simulink model "B4CostaTest"  (R2022a)
settings: Solver=VariableStepAuto  StartTime=0.0  StopTime=40  RelTol=1e-4  AbsTol=1e-4
values from neighbouring files (symbols this model uses):
  AinfK_h_B4 = -23    [B4.m]
  AinfK_p_B4 = 1.0    (= 1)    [B4.m]
  AinfK_s_B4 = 9.0    (= 9)    [B4.m]
  AinfNa_h_B4 = -37    [B4.m]
  AinfNa_p_B4 = 1.0    (= 1)    [B4.m]
  AinfNa_s_B4 = 5.0    (= 5)    [B4.m]
  AK_B4_0 = 0.4    [B4.m]
  ANa_B4_0 = 0.4    [B4.m]
  BinfNa_h_B4 = -43.0    (= -43)    [B4.m]
  BinfNa_p_B4 = 1.0    (= 1)    [B4.m]
  BinfNa_s_B4 = 5.0    (= 5)    [B4.m]
  BNa_B4_0 = 0.4    [B4.m]
  Cm_B4 = 0.01    [B4.m]    (also in CtrlParaSNSTuning.m)
  EK_B4 = -70    [B4.m]
  EL_B4 = -60    [B4.m]    (also in CtrlParaSNSTuning.m)
  ENa_B4 = 30    [B4.m]
  gK_B4 = 12    [B4.m]
  gL_B4 = 0.1    [B4.m]    (also in CtrlParaSNSTuning.m = 0.2008)
  gNa_B4 = 25    [B4.m]
  pK_B4 = 4    [B4.m]
  pNa_B4 = 3    [B4.m]
  RK_B4 = 0    [B4.m]
  RL_B4 = 0    [B4.m]    (also in CtrlParaSNSTuning.m)
  RNa_B4 = 0    [B4.m]
  spikedur_B4 = 0.003    [B4.m]
  tAK_h_B4 = -8.0    (= -8)    [B4.m]
  tAK_p_B4 = 1.0    (= 1)    [B4.m]
  tAK_s_B4 = 10.0    (= 10)    [B4.m]
  tAK_tmax_B4 = 0.04    [B4.m]
  tAK_tmin_B4 = 0.004    [B4.m]
  tANa_h_B4 = -43    [B4.m]
  tANa_p_B4 = 1.0    (= 1)    [B4.m]
  tANa_s_B4 = 4.0    (= 4)    [B4.m]
  tANa_tmax_B4 = 0.006    [B4.m]
  tANa_tmin_B4 = 0.001    [B4.m]
  tBNa_h_B4 = -38    [B4.m]
  tBNa_p_B4 = 1.0    (= 1)    [B4.m]
  tBNa_s_B4 = 10.0    (= 10)    [B4.m]
  tBNa_tmax_B4 = 0.02    [B4.m]
  tBNa_tmin_B4 = 0.005    [B4.m]
  V_B4_0 = -60    [B4.m]    (also in CtrlParaSNSTuning.m; InitPara.m)
undefined symbols (not defined in the file or in its folder): Iapp
libraries: simulink x1
settings Model: Creator=liyan  LastModifiedBy=liyan

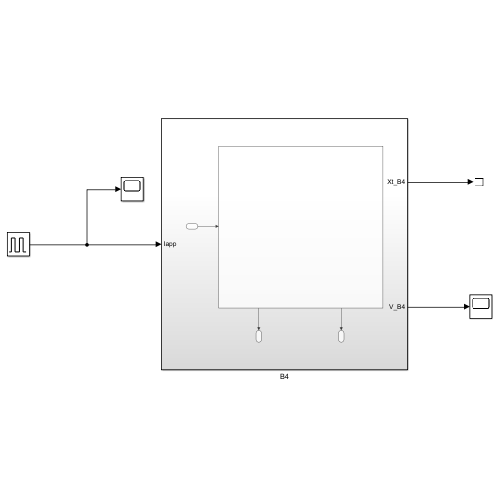
[thumbnail: Simulink's stored preview of the top-level diagram]
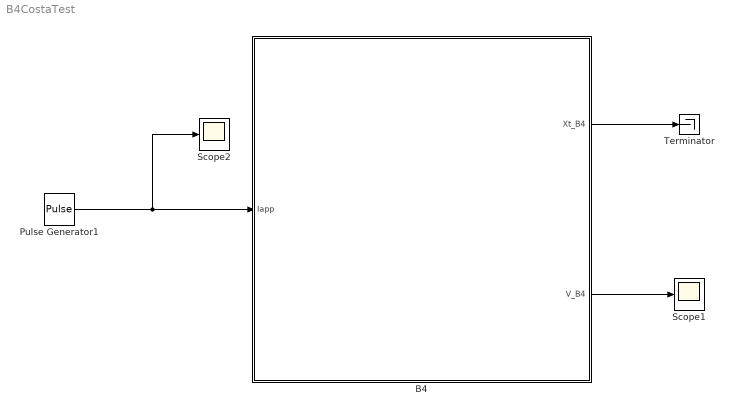
== system B4CostaTest ==
  B4 : Subsystem
  Pulse Generator1 : DiscretePulseGenerator  PulseType=Time based  Amplitude=Iapp  Period=40  PulseWidth=0.3/40*100  PhaseDelay=30
  Scope1 : Scope
  Scope2 : Scope
  Terminator : Terminator
  wires:
  Pulse Generator1/1 -> B4/1(Iapp), Scope2/1
  B4/2(V_B4) -> Scope1/1
  B4/1(Xt_B4) -> Terminator/1

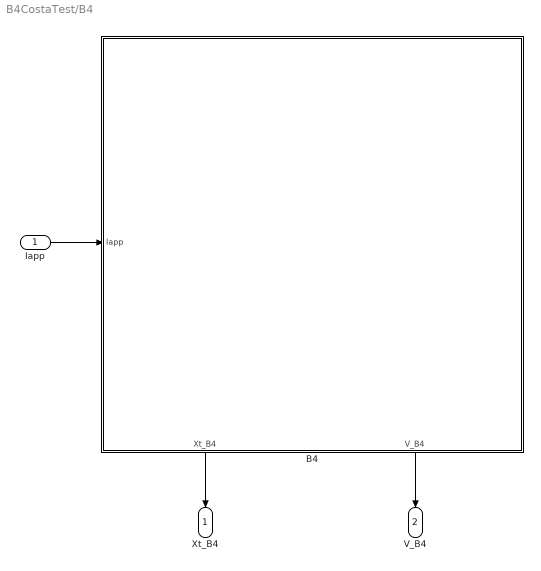
== system B4CostaTest/B4 ==
  Iapp : Inport
  B4 : Subsystem
      settings: PortSchema="{\"entries\":[{\"content\":{\"sides\":[{\"content\":{\"connectorIds\":[\"In1\"]},\"type\":\"ConnectorPlacement.EquallySpacedRectSide\",\"uuid\":\"24c72156-30eb-49cf-b194-b2525f55826e\"},{\"content\":{\"connectorIds\":[],\"side\":\"RIGHT\"},\"type\":\"ConnectorPlacement.EquallySpacedRectSide\",\"uuid\":\"58ba20b4-fd31-4cee-a6c8-4543f1171f3d\"},{\"content\":{\"connectorIds\":[\"Out1\",\"Out2\"],\"side\":\"TOP\"},\"type\":\"ConnectorPlacement.EquallySpacedRectSide\",\"uuid\":\"5721a781-56a7-44d1-83f7-f714f73d5f12\"},{\"content\":{\"connectorIds\":[],\"side\":\"BOTTOM\"},\"type\":\"ConnectorPlacement.EquallySpacedRectSide\",\"uuid\":\"82e70541-a058-4704-89bd-0c8445a0faee\"}]},\"type\":\"ConnectorPlacement.EquallySpacedConnector\",\"uuid\":\"3f261af1-2108-4b15-8c2d-24b61f10e15a\"}],\"packageUris\":[\"http://schema.mathworks.com/mf0/Connector/R2020b\"],\"version\":\"1.0\"}"
  Xt_B4 : Outport
  V_B4 : Outport  Port=2
  wires:
  B4/1(Xt_B4) -> Xt_B4/1
  Iapp/1 -> B4/1(Iapp)
  B4/2(V_B4) -> V_B4/1

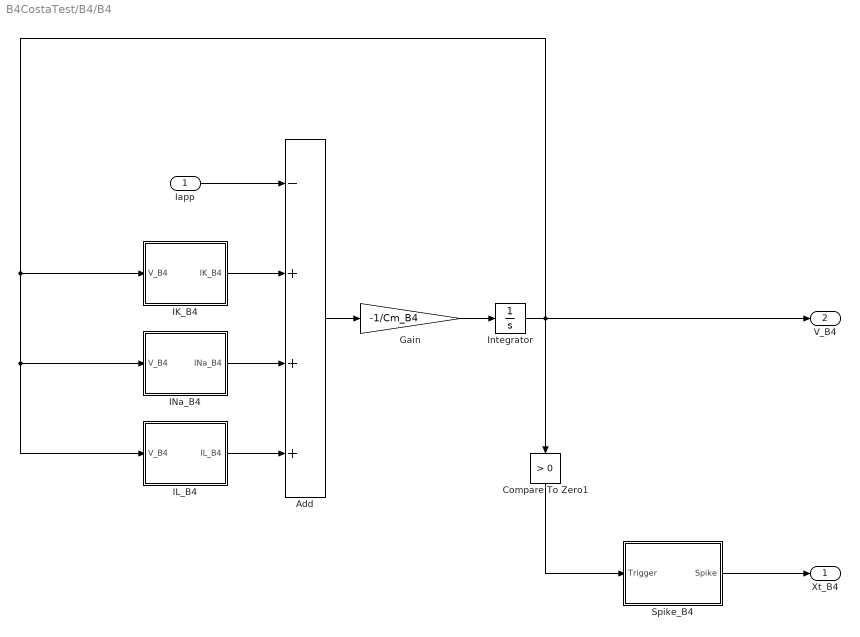
== system B4CostaTest/B4/B4 ==
  Iapp : Inport
  Add : Sum  Inputs=-+++
  Compare To Zero1 : simulink/Logic and Bit Operations/Compare To Zero  relop=>  OutDataTypeStr=boolean
  Gain : Gain  Gain=-1/Cm_B4
  IK_B4 : Subsystem
  IL_B4 : Subsystem
  INa_B4 : Subsystem
  Integrator : Integrator  InitialCondition=V_B4_0
  Spike_B4 : Subsystem
  Xt_B4 : Outport
  V_B4 : Outport  Port=2
  wires:
  Gain/1 -> Integrator/1
  Add/1 -> Gain/1
  Compare To Zero1/1 -> Spike_B4/1(Trigger)
  Spike_B4/1(Spike) -> Xt_B4/1
  Integrator/1 -> V_B4/1, Compare To Zero1/1, IK_B4/1(V_B4), INa_B4/1(V_B4), IL_B4/1(V_B4)
  Iapp/1 -> Add/1
  IK_B4/1(IK_B4) -> Add/2
  INa_B4/1(INa_B4) -> Add/3
  IL_B4/1(IL_B4) -> Add/4

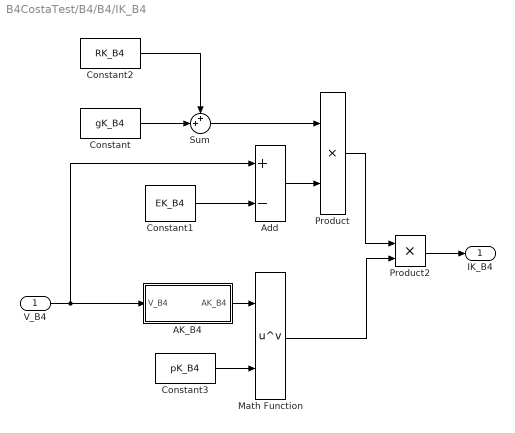
== system B4CostaTest/B4/B4/IK_B4 ==
  V_B4 : Inport
  AK_B4 : Subsystem
  Add : Sum  Inputs=+-
  Constant : Constant  Value=gK_B4
  Constant1 : Constant  Value=EK_B4
  Constant2 : Constant  Value=RK_B4
  Constant3 : Constant  Value=pK_B4
  Math Function : Math  Operator=pow
  Product : Product
  Product2 : Product
  Sum : Sum  Inputs=++|
  IK_B4 : Outport
  wires:
  Add/1 -> Product/2
  Constant1/1 -> Add/2
  V_B4/1 -> AK_B4/1(V_B4), Add/1
  Product/1 -> Product2/1
  Math Function/1 -> Product2/2
  Product2/1 -> IK_B4/1
  Constant/1 -> Sum/2
  Sum/1 -> Product/1
  Constant2/1 -> Sum/1
  AK_B4/1(AK_B4) -> Math Function/1
  Constant3/1 -> Math Function/2

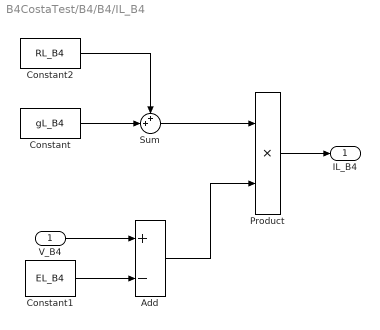
== system B4CostaTest/B4/B4/IL_B4 ==
  V_B4 : Inport
  Add : Sum  Inputs=+-
  Constant : Constant  Value=gL_B4
  Constant1 : Constant  Value=EL_B4
  Constant2 : Constant  Value=RL_B4
  Product : Product
  Sum : Sum  Inputs=++|
  IL_B4 : Outport
  wires:
  Constant1/1 -> Add/2
  V_B4/1 -> Add/1
  Constant2/1 -> Sum/1
  Sum/1 -> Product/1
  Constant/1 -> Sum/2
  Add/1 -> Product/2
  Product/1 -> IL_B4/1

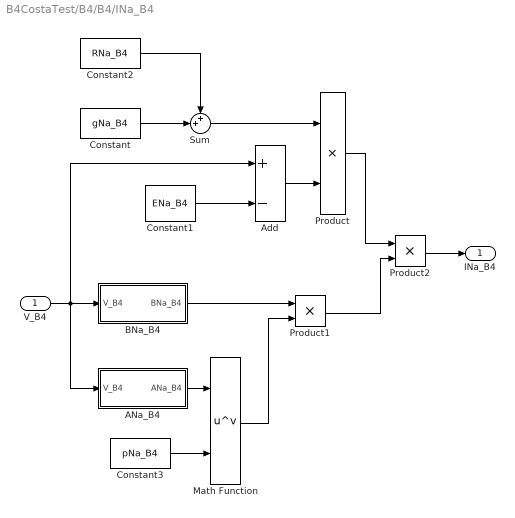
== system B4CostaTest/B4/B4/INa_B4 ==
  V_B4 : Inport
  ANa_B4 : Subsystem
  Add : Sum  Inputs=+-
  BNa_B4 : Subsystem
  Constant : Constant  Value=gNa_B4
  Constant1 : Constant  Value=ENa_B4
  Constant2 : Constant  Value=RNa_B4
  Constant3 : Constant  Value=pNa_B4
  Math Function : Math  Operator=pow
  Product : Product
  Product1 : Product
  Product2 : Product
  Sum : Sum  Inputs=++|
  INa_B4 : Outport
  wires:
  Add/1 -> Product/2
  Constant1/1 -> Add/2
  V_B4/1 -> ANa_B4/1(V_B4), BNa_B4/1(V_B4), Add/1
  Product/1 -> Product2/1
  Product1/1 -> Product2/2
  Product2/1 -> INa_B4/1
  Constant/1 -> Sum/2
  Sum/1 -> Product/1
  Constant2/1 -> Sum/1
  ANa_B4/1(ANa_B4) -> Math Function/1
  Constant3/1 -> Math Function/2
  BNa_B4/1(BNa_B4) -> Product1/1
  Math Function/1 -> Product1/2

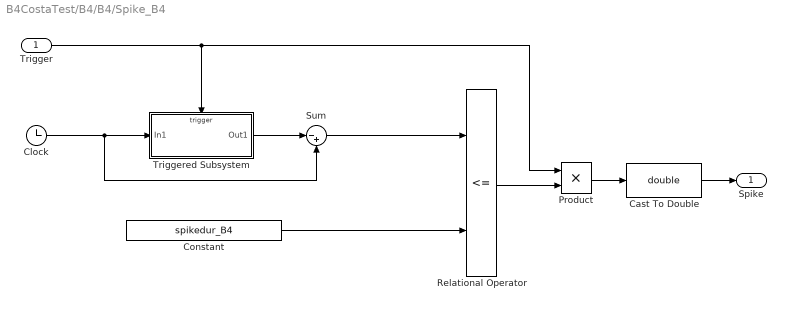
== system B4CostaTest/B4/B4/Spike_B4 ==
  Trigger : Inport
  Cast To Double : DataTypeConversion  OutDataTypeStr=double  SaturateOnIntegerOverflow=off  RndMeth=Floor
  Clock : Clock
  Constant : Constant  Value=spikedur_B4
  Product : Product
  Relational Operator : RelationalOperator  Operator=<=  OutDataTypeStr=boolean  RndMeth=Simplest  InputSameDT=off
  Sum : Sum  Inputs=|-+
  Triggered Subsystem : Subsystem  TreatAsAtomicUnit=on
  Spike : Outport
  wires:
  Clock/1 -> Sum/2, Triggered Subsystem/1(In1)
  Triggered Subsystem/1(Out1) -> Sum/1
  Constant/1 -> Relational Operator/2
  Trigger/1 -> Triggered Subsystem/Trigger, Product/1
  Sum/1 -> Relational Operator/1
  Relational Operator/1 -> Product/2
  Product/1 -> Cast To Double/1
  Cast To Double/1 -> Spike/1

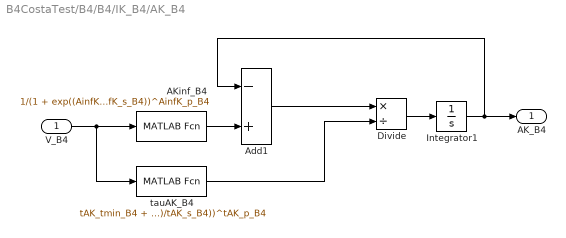
== system B4CostaTest/B4/B4/IK_B4/AK_B4 ==
  V_B4 : Inport
  AKinf_B4 : MATLABFcn  MATLABFcn=1/(1 + exp((AinfK_h_B4 - u(1))/AinfK_s_B4))^AinfK_p_B4
  Add1 : Sum  Inputs=-+
  Divide : Product  Inputs=*/
  Integrator1 : Integrator  InitialCondition=AK_B4_0
  tauAK_B4 : MATLABFcn  MATLABFcn=tAK_tmin_B4 + (tAK_tmax_B4 - tAK_tmin_B4)/(1 + exp((u(1) - tAK_h_B4)/tAK_s_B4))^tAK_p_B4
  AK_B4 : Outport
  wires:
  tauAK_B4/1 -> Divide/2
  Divide/1 -> Integrator1/1
  V_B4/1 -> tauAK_B4/1, AKinf_B4/1
  Integrator1/1 -> Add1/1, AK_B4/1
  Add1/1 -> Divide/1
  AKinf_B4/1 -> Add1/2

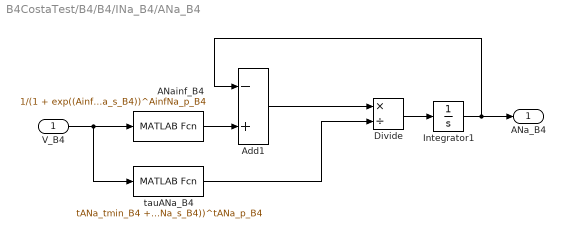
== system B4CostaTest/B4/B4/INa_B4/ANa_B4 ==
  V_B4 : Inport
  ANainf_B4 : MATLABFcn  MATLABFcn=1/(1 + exp((AinfNa_h_B4 - u(1))/AinfNa_s_B4))^AinfNa_p_B4
  Add1 : Sum  Inputs=-+
  Divide : Product  Inputs=*/
  Integrator1 : Integrator  InitialCondition=ANa_B4_0
  tauANa_B4 : MATLABFcn  MATLABFcn=tANa_tmin_B4 + (tANa_tmax_B4 - tANa_tmin_B4)/(1 + exp((u(1) - tANa_h_B4)/tANa_s_B4))^tANa_p_B4
  ANa_B4 : Outport
  wires:
  tauANa_B4/1 -> Divide/2
  Divide/1 -> Integrator1/1
  V_B4/1 -> tauANa_B4/1, ANainf_B4/1
  Integrator1/1 -> Add1/1, ANa_B4/1
  Add1/1 -> Divide/1
  ANainf_B4/1 -> Add1/2

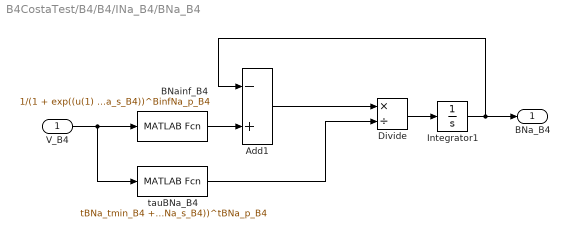
== system B4CostaTest/B4/B4/INa_B4/BNa_B4 ==
  V_B4 : Inport
  Add1 : Sum  Inputs=-+
  BNainf_B4 : MATLABFcn  MATLABFcn=1/(1 + exp((u(1) - BinfNa_h_B4)/BinfNa_s_B4))^BinfNa_p_B4
  Divide : Product  Inputs=*/
  Integrator1 : Integrator  InitialCondition=BNa_B4_0
  tauBNa_B4 : MATLABFcn  MATLABFcn=tBNa_tmin_B4 + (tBNa_tmax_B4 - tBNa_tmin_B4)/(1 + exp((u(1) - tBNa_h_B4)/tBNa_s_B4))^tBNa_p_B4
  BNa_B4 : Outport
  wires:
  tauBNa_B4/1 -> Divide/2
  Divide/1 -> Integrator1/1
  V_B4/1 -> tauBNa_B4/1, BNainf_B4/1
  Integrator1/1 -> Add1/1, BNa_B4/1
  Add1/1 -> Divide/1
  BNainf_B4/1 -> Add1/2

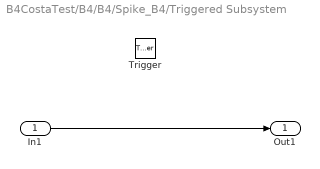
== system B4CostaTest/B4/B4/Spike_B4/Triggered Subsystem ==
  In1 : Inport
  Trigger : TriggerPort  VariantControl=Variant
  Out1 : Outport
  wires:
  In1/1 -> Out1/1
